simulink model "test"  (R2020b)
settings: Solver=ode4  StartTime=0.0  StopTime=10  FixedStep=0.001  RelTol=1e-3
settings Model: Creator=tian  LastModifiedBy=tian

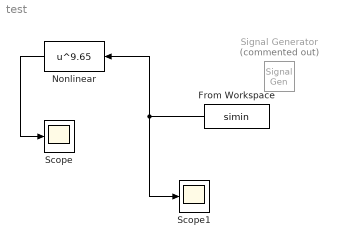
== system test ==
  From Workspace : FromWorkspace  VariableName=simin
  Nonlinear : Fcn  Expr=u^9.65
  Scope : Scope
  Scope1 : Scope
  Signal Generator : SignalGenerator  Commented=on  Amplitude=0.9
  wires:
  Nonlinear/1 -> Scope/1
  From Workspace/1 -> Scope1/1, Nonlinear/1
